simulink model "exerc2_blocks"  (R2022a)
settings: Solver=VariableStepAuto  StartTime=0.0  StopTime=10  RelTol=1e-3
values from neighbouring files (symbols this model uses):
  beta = 20/N    (= 10)    [exerc2.m]
  g = 9.8    [exerc2.m]
  J_m = N    (= 2)    [exerc2.m]
  k_b = 0.1*N    (= 0.2)    [exerc2.m]
  k_i = 20/N    (= 10)    [exerc2.m]
  L = N    (= 2)    [exerc2.m]
  L_a = 0.1*N    (= 0.2)    [exerc2.m]
  m = sqrt(1/N)    [exerc2.m]
  R_a = 20/N    (= 10)    [exerc2.m]
  x_0 = [x1_0 x2_0 x3_0]    [exerc1.m]    (also in exerc2.m = 0.5)
libraries: slpidlib x1
settings Model: Creator=marbian  LastModifiedBy=marbian

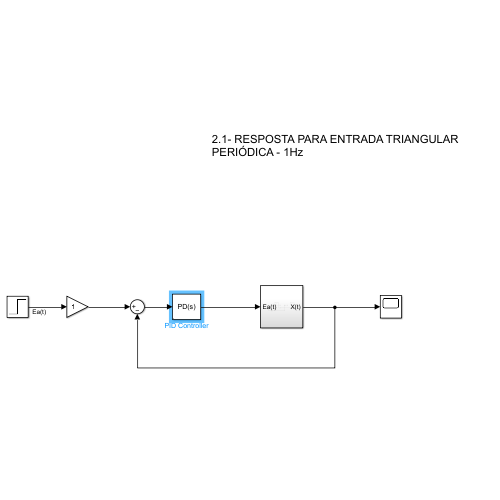
[thumbnail: Simulink's stored preview of the top-level diagram]
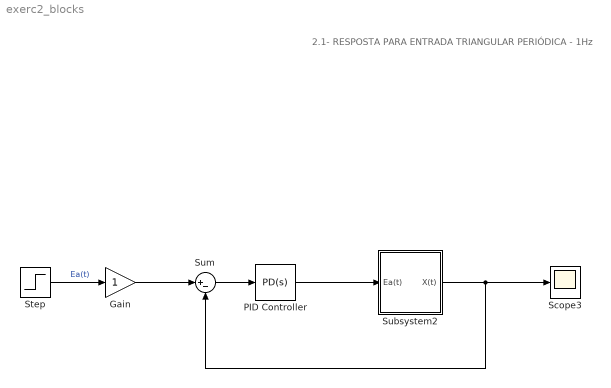
== system exerc2_blocks ==
  note: 2.1- RESPOSTA PARA ENTRADA TRIANGULAR PERIÓDICA - 1Hz
  Gain : Gain
  PID Controller : slpidlib/PID Controller  Controller=PD  Form=Parallel  TimeDomain=Continuous-time  UseExternalTs=off  SampleTime=-1  IntegratorMethod=Forward Euler  FilterMethod=Forward Euler  ControllerParametersSource=internal  P=22.9507493762383  I=1  UseKiTs=off  D=8.12106683086206  N=2.04910341628753  UseFilter=on  TunerSelectOption=Transfer Function Based (PID Tuner App)  InitialConditionSource=internal  InitialConditionForIntegrator=0  InitialConditionForFilter=0  DifferentiatorICPrevScaledInput=0  ExternalReset=none  TrackingMode=off  Kt=1  LimitOutput=off  SatLimitsSource=internal  UpperSaturationLimit=inf  LowerSaturationLimit=-inf  LinearizeAsGain=on  AntiWindupMode=none  Kb=1  POutMin=[]  POutMax=[]  IOutMin=[]  IOutMax=[]  DOutMin=[]  DOutMax=[]  NOutMin=[]  NOutMax=[]  SumOutMin=[]  SumOutMax=[]  SaturationOutMin=[]  SaturationOutMax=[]  PParamMin=[]  PParamMax=[]  IParamMin=[]  IParamMax=[]  DParamMin=[]  DParamMax=[]  NParamMin=[]  NParamMax=[]  KbParamMin=[]  KbParamMax=[]  KtParamMin=[]  KtParamMax=[]  KbOutMin=[]  KbOutMax=[]  KtOutMin=[]  KtOutMax=[]  IntegratorOutMin=[]  IntegratorOutMax=[]  FilterOutMin=[]  FilterOutMax=[]  SumI1OutMin=[]  SumI1OutMax=[]  SumI2OutMin=[]  SumI2OutMax=[]  SumI3OutMin=[]  SumI3OutMax=[]  SumI4OutMin=[]  SumI4OutMax=[]  SumDOutMin=[]  SumDOutMax=[]  DifferentiatorOutMin=[]  DifferentiatorOutMax=[]  FilterDiffOutCoefMin=[]  FilterDiffOutCoefMax=[]  ReciprocalOutMin=[]  ReciprocalOutMax=[]  SumDenOutMin=[]  SumDenOutMax=[]  SumNumOutMin=[]  SumNumOutMax=[]  DivideOutMin=[]  DivideOutMax=[]  UdiffTsProdOutMin=[]  UdiffTsProdOutMax=[]  NTsProdOutMin=[]  NTsProdOutMax=[]  UintegralTsProdOutMin=[]  UintegralTsProdOutMax=[]  UngainTsProdOutMin=[]  UngainTsProdOutMax=[]  IntegratorContinuousStateAttributes=''  IntegratorStateMustResolveToSignalObject=off  IntegratorRTWStateStorageClass=Auto  FilterContinuousStateAttributes=''  FilterStateMustResolveToSignalObject=off  FilterRTWStateStorageClass=Auto  ParallelPVariant=InternalParameters  IdealPVariant=Disabled  IVariant=Disabled  DVariant=InternalParameters  IntegratorVariant=Disabled  SatVariant=Disabled  AWVariant=Disabled  PCopyVariant=Disabled  TRVariant=Disabled  FdbkBlocksVariant=Forward  IdealPFdbkVariant=Disabled  SatFdbkVariant=Disabled  DerivativeFilterVariant=ContFilter  NVariant=InternalParameters  NCopyVariant=Disabled  FilterICVariant=InternalICsFilter  IntegratorICVariant=Disabled  ExternalResetVariant=Disabled  TRSumVariant=Passthrough  SumFdbkVariant=Disabled  SumVariant=Sum_PD  TsampFilterVariant=InternalTs  TsampNgainVariant=Passthrough  TsampIntegralVariant=Disabled_SignalSpec  ExternalSaturationOutDataTypeStr=Inherit: Same as second input  aMode=0
  Scope3 : Scope
  Step : Step  SampleTime=0
  Subsystem2 : Subsystem
  Sum : Sum  Inputs=|+-
  wires:
  Subsystem2/1(X(t)) -> Sum/2, Scope3/1
  PID Controller/1 -> Subsystem2/1(Ea(t))
  Sum/1 -> PID Controller/1
  Gain/1 -> Sum/1
  Step/1 -> Gain/1  "Ea(t)"

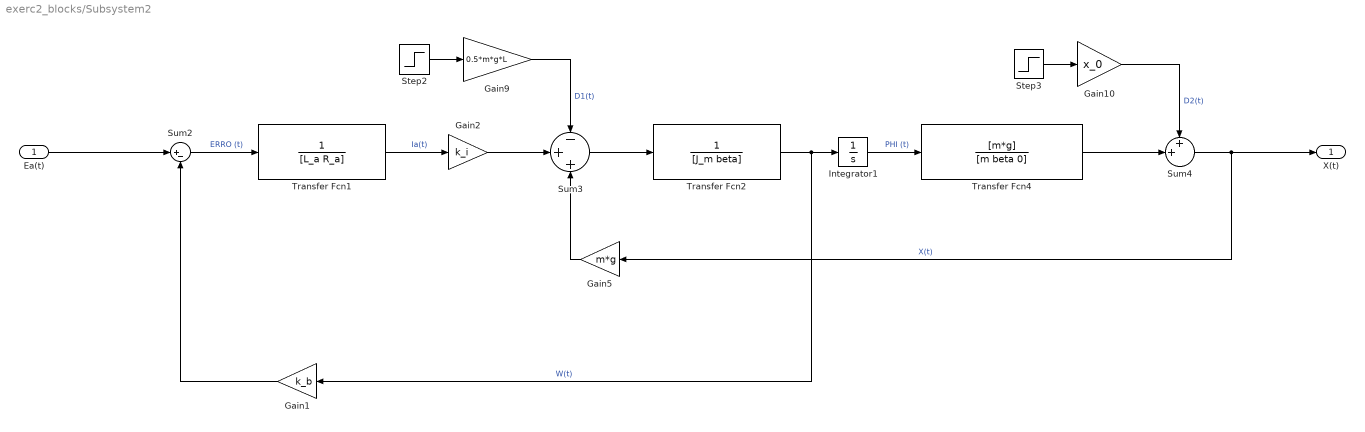
== system exerc2_blocks/Subsystem2 ==
  Ea(t) : Inport
  Gain1 : Gain  Gain=k_b
  Gain10 : Gain  Gain=x_0
  Gain2 : Gain  Gain=k_i
  Gain5 : Gain  Gain=m*g
  Gain9 : Gain  Gain=0.5*m*g*L
  Integrator1 : Integrator
  Step2 : Step  Time=0  SampleTime=0
  Step3 : Step  Time=0  SampleTime=0
  Sum2 : Sum  Inputs=|+-
  Sum3 : Sum  Inputs=-++
  Sum4 : Sum  Inputs=++|
  Transfer Fcn1 : TransferFcn  Denominator=[L_a R_a]
  Transfer Fcn2 : TransferFcn  Denominator=[J_m beta]
  Transfer Fcn4 : TransferFcn  Numerator=[m*g]  Denominator=[m beta 0]
  X(t) : Outport
  wires:
  Gain1/1 -> Sum2/2
  Transfer Fcn2/1 -> Gain1/1, Integrator1/1  "W(t)"
  Sum4/1 -> X(t)/1, Gain5/1  "X(t)"
  Gain5/1 -> Sum3/3
  Integrator1/1 -> Transfer Fcn4/1  "PHI (t)"
  Sum2/1 -> Transfer Fcn1/1  "ERRO (t)"
  Transfer Fcn4/1 -> Sum4/2
  Sum3/1 -> Transfer Fcn2/1
  Step2/1 -> Gain9/1
  Gain9/1 -> Sum3/1  "D1(t)"
  Gain2/1 -> Sum3/2
  Gain10/1 -> Sum4/1  "D2(t)"
  Transfer Fcn1/1 -> Gain2/1  "Ia(t)"
  Ea(t)/1 -> Sum2/1
  Step3/1 -> Gain10/1
